simulink model "twsbr_plant"  (R2026a)
settings: Solver=ode45  StopTime=2.0  MaxStep=0.01  RelTol=1e-9  AbsTol=1e-11
settings Model: Creator=Linxiuqi  LastModifiedBy=Linxiuqi

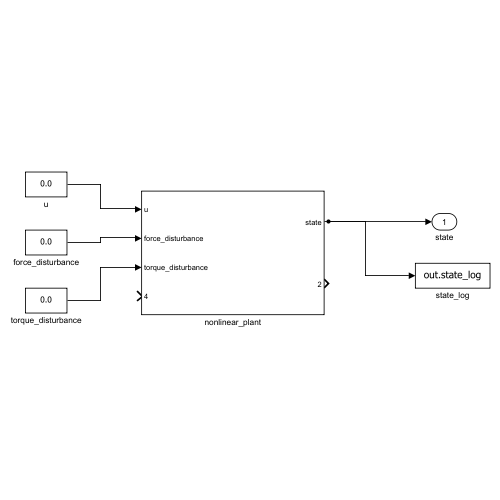
[thumbnail: Simulink's stored preview of the top-level diagram]
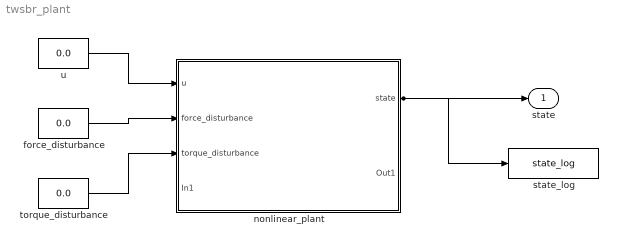
== system twsbr_plant ==
  force_disturbance : Constant  Value=0.0
  nonlinear_plant : Subsystem
  state_log : ToWorkspace  VariableName=state_log  SaveFormat=Structure With Time  SampleTime=-1
  torque_disturbance : Constant  Value=0.0
  u : Constant  Value=0.0
  state : Outport
  wires:
  u/1 -> nonlinear_plant/1(u)
  force_disturbance/1 -> nonlinear_plant/2(force_disturbance)
  torque_disturbance/1 -> nonlinear_plant/3(torque_disturbance)
  nonlinear_plant/1(state) -> state/1, state_log/1

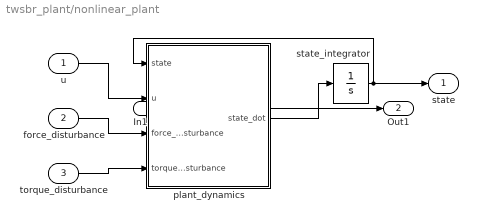
== system twsbr_plant/nonlinear_plant ==
  u : Inport
  force_disturbance : Inport  Port=2
  torque_disturbance : Inport  Port=3
  In1 : Inport  Port=4
  plant_dynamics : MATLAB Function  TreatAsAtomicUnit=on
  state_integrator : Integrator  InitialCondition=[0;0;0;0]
  state : Outport
  Out1 : Outport  Port=2
  wires:
  In1/1 -> Out1/1
  state_integrator/1 -> plant_dynamics/1(state), state/1
  u/1 -> plant_dynamics/2(u)
  force_disturbance/1 -> plant_dynamics/3(force_disturbance)
  torque_disturbance/1 -> plant_dynamics/4(torque_disturbance)
  plant_dynamics/1(state_dot) -> state_integrator/1

== matlab function twsbr_plant/nonlinear_plant/plant_dynamics ==
  data: state input; u input; state_dot output; force_disturbance input; torque_disturbance input
function state_dot = plant_dynamics(state, u, force_disturbance, torque_disturbance)
%#codegen
body_mass = 1.2;
wheel_mass = 0.29999999999999999;
com_length = 0.17999999999999999;
body_inertia = 0.025000000000000001;
damping = 0.050000000000000003;
gravity = 9.8100000000000005;
motor_gain = 12;
x_dot = state(2);
theta = state(3);
theta_dot = state(4);
force = motor_gain * u + force_disturbance;
mass_sum = wheel_mass + body_mass;
rotational_term = body_inertia + body_mass * com_length^2;
coupling = body_mass * com_length * cos(theta);
rhs_position = force - damping * x_dot + body_mass * com_length * theta_dot^2 * sin(theta);
rhs_angle = body_mass * gravity * com_length * sin(theta) + torque_disturbance;
determinant = mass_sum * rotational_term - coupling^2;
x_ddot = (rotational_term * rhs_position - coupling * rhs_angle) / determinant;
theta_ddot = (-coupling * rhs_position + mass_sum * rhs_angle) / determinant;
state_dot = [x_dot; x_ddot; theta_dot; theta_ddot];
end
